simulink model "gm_RNN_Node"  (R2020b)
settings: Solver=VariableStepAuto  StartTime=0.0  StopTime=10.0  RelTol=1e-3
libraries: hdlmdlgenlib x1
settings Model: Creator=chank  LastModifiedBy=chank
settings OptimizationCC: BlockReduction=off  ConditionallyExecuteInputs=off
settings DebuggingCC: InheritedTsInSrcMsg=none

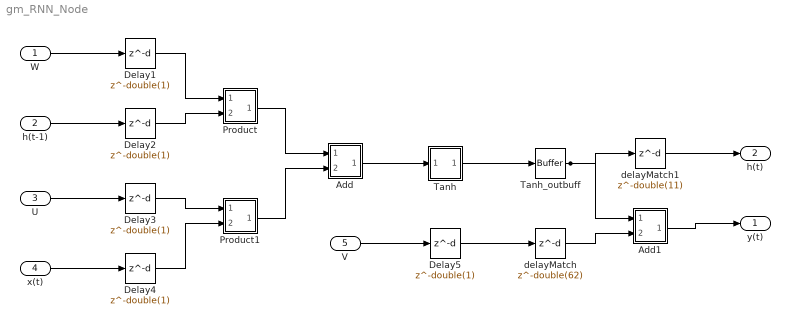
== system gm_RNN_Node ==
  W : Inport  OutDataTypeStr=single  PortDimensions=1  SampleTime=0.2
  h(t-1) : Inport  Port=2  OutDataTypeStr=single  PortDimensions=1  SampleTime=0.2
  U : Inport  Port=3  OutDataTypeStr=single  PortDimensions=1  SampleTime=0.2
  x(t) : Inport  Port=4  OutDataTypeStr=single  PortDimensions=1  SampleTime=0.2
  V : Inport  Port=5  OutDataTypeStr=single  PortDimensions=1  SampleTime=0.2
  Add : Subsystem
      mask Display: disp('NFP\nadd');
  Add1 : Subsystem
      mask Display: disp('NFP\nadd');
  Delay{1..5} (5 alike) : Delay  DelayLength=double(1)  InitialCondition=0  SampleTime=0.2
  Product : Subsystem
      mask Display: disp('NFP\nmul');
  Product1 : Subsystem
      mask Display: disp('NFP\nmul');
  Tanh : Subsystem
      mask Display: disp('NFP\ntrig');
  Tanh_outbuff : hdlmdlgenlib/Buffer
      settings: SourceProductBaseCode=SL
  delayMatch : Delay  DelayLength=double(62)  InitialCondition=0  SampleTime=0.2
  delayMatch1 : Delay  DelayLength=double(11)  InitialCondition=0  SampleTime=0.2
  y(t) : Outport
  h(t) : Outport  Port=2
  wires:
  W/1 -> Delay1/1
  h(t-1)/1 -> Delay2/1
  U/1 -> Delay3/1
  x(t)/1 -> Delay4/1
  V/1 -> Delay5/1
  Delay1/1 -> Product/1(In1)
  Delay2/1 -> Product/2(In2)
  Delay3/1 -> Product1/1(In1)
  Delay4/1 -> Product1/2(In2)
  delayMatch/1 -> Add1/2(In2)
  delayMatch1/1 -> h(t)/1
  Add/1(Out1) -> Tanh/1(In1)
  Add1/1(Out1) -> y(t)/1
  Product/1(Out1) -> Add/1(In1)
  Product1/1(Out1) -> Add/2(In2)
  Tanh/1(Out1) -> Tanh_outbuff/1
  Delay5/1 -> delayMatch/1
  Tanh_outbuff/1 -> delayMatch1/1, Add1/1(In1)

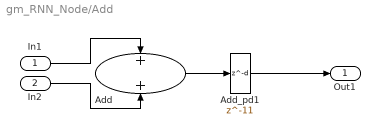
== system gm_RNN_Node/Add ==
  In1 : Inport
  In2 : Inport  Port=2
  Add : Sum  OutDataTypeStr=single  SampleTime=0.2
  Add_pd1 : Delay  DelayLength=11
  Out1 : Outport
  wires:
  In1/1 -> Add/1
  In2/1 -> Add/2
  Add/1 -> Add_pd1/1
  Add_pd1/1 -> Out1/1

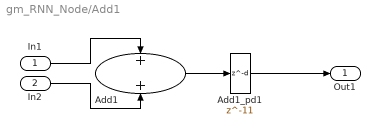
== system gm_RNN_Node/Add1 ==
  In1 : Inport
  In2 : Inport  Port=2
  Add1 : Sum  OutDataTypeStr=single  SampleTime=0.2
  Add1_pd1 : Delay  DelayLength=11
  Out1 : Outport
  wires:
  In1/1 -> Add1/1
  In2/1 -> Add1/2
  Add1/1 -> Add1_pd1/1
  Add1_pd1/1 -> Out1/1

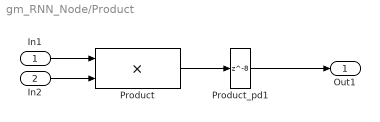
== system gm_RNN_Node/Product ==
  In1 : Inport
  In2 : Inport  Port=2
  Product : Product  Inputs=**  OutDataTypeStr=single  SampleTime=0.2
  Product_pd1 : Delay  DelayLength=8
  Out1 : Outport
  wires:
  In1/1 -> Product/1
  In2/1 -> Product/2
  Product/1 -> Product_pd1/1
  Product_pd1/1 -> Out1/1

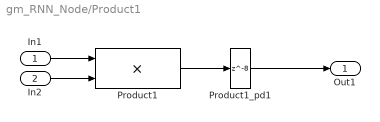
== system gm_RNN_Node/Product1 ==
  In1 : Inport
  In2 : Inport  Port=2
  Product1 : Product  Inputs=**  OutDataTypeStr=single  SampleTime=0.2
  Product1_pd1 : Delay  DelayLength=8
  Out1 : Outport
  wires:
  In1/1 -> Product1/1
  In2/1 -> Product1/2
  Product1/1 -> Product1_pd1/1
  Product1_pd1/1 -> Out1/1

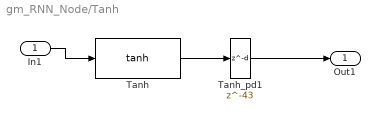
== system gm_RNN_Node/Tanh ==
  In1 : Inport
  Tanh : Trigonometry  Operator=tanh  SampleTime=0.2
  Tanh_pd1 : Delay  DelayLength=43
  Out1 : Outport
  wires:
  In1/1 -> Tanh/1
  Tanh/1 -> Tanh_pd1/1
  Tanh_pd1/1 -> Out1/1
